simulink model "PhysicalHyperCook"  (R2026b)
settings: Solver=VariableStepAuto  StopTime=14400
undefined symbols (not defined in the file): Fault_T_Cook1, Fault_T_Cook2, Fault_T_Cook3, Fault_T_Cook4, Fault_T_Pack, Fault_T_Prep1, Fault_T_Prep2, Fault_T_QC, HC_PackRate_bph, HC_PrepRate_bph, HC_QCRate_bph, HC_Resupply_bph, Recipe_Block_s, Recipe_Count, Recipe_Flush_s, Resupply_Cutoff_T, Transport_Latency_s, Transport_Rate_bph
(part 2 of 2)

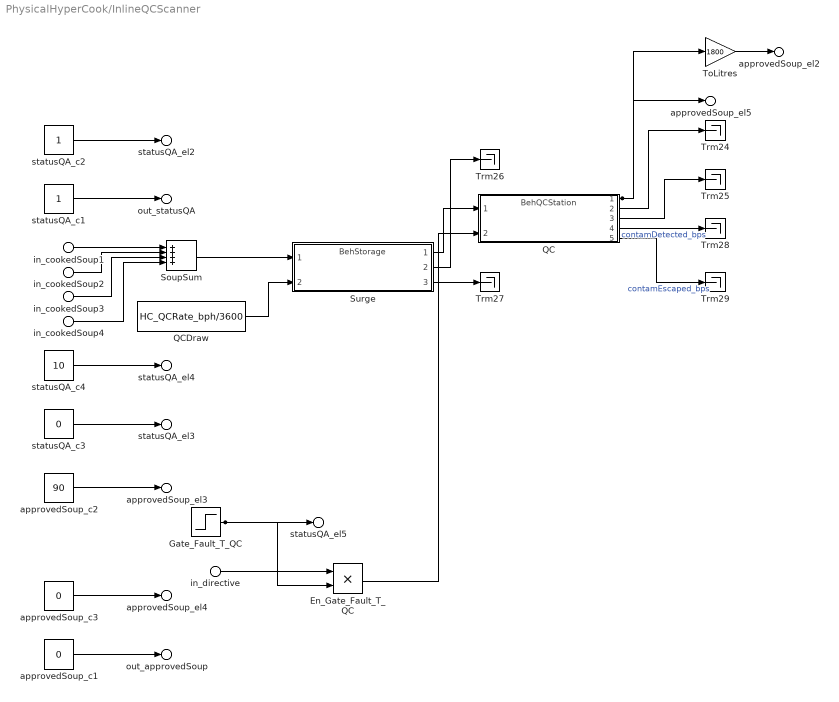
== system PhysicalHyperCook/InlineQCScanner ==
  in_cookedSoup1 : Inport  PortName=cookedSoup1  Element=flow_bps
  in_cookedSoup2 : Inport  Port=2  PortName=cookedSoup2  Element=flow_bps
  in_cookedSoup3 : Inport  Port=3  PortName=cookedSoup3  Element=flow_bps
  in_cookedSoup4 : Inport  Port=4  PortName=cookedSoup4  Element=flow_bps
  in_directive : Inport  Port=5  PortName=directive  Element=setpoint
  En_Gate_Fault_T_QC : Product
  Gate_Fault_T_QC : Step  Time=Fault_T_QC  InitialValue=1  FinalValue=0  SampleTime=0
  QC : ModelReference  ModelNameDialog=BehQCStation  UsingDefaultArgumentValue=0,0,0,0,0,0  SimulationMode=Normal  ModelReferenceVersion=1.6
  QCDraw : Constant  Value=HC_QCRate_bph/3600
  SoupSum : Sum  Inputs=++++
  Surge : ModelReference  ModelNameDialog=BehStorage  UsingDefaultArgumentValue=0,0  SimulationMode=Normal  ModelReferenceVersion=1.4
  ToLitres : Gain  Gain=1800
  Trm{24..29} (6 alike) : Terminator
  approvedSoup_c1 : Constant  Value=0
  approvedSoup_c2 : Constant  Value=90
  approvedSoup_c3 : Constant  Value=0
  statusQA_c1 : Constant
  statusQA_c2 : Constant
  statusQA_c3 : Constant  Value=0
  statusQA_c4 : Constant  Value=10
  out_approvedSoup : Outport  PortName=approvedSoup  Element=batchId
  approvedSoup_el2 : Outport  PortName=approvedSoup  Element=volume_L
  approvedSoup_el3 : Outport  PortName=approvedSoup  Element=temp_C
  approvedSoup_el4 : Outport  PortName=approvedSoup  Element=contamination_ppm
  approvedSoup_el5 : Outport  PortName=approvedSoup  Element=flow_bps
  out_statusQA : Outport  Port=2  PortName=statusQA  Element=unitId
  statusQA_el2 : Outport  Port=2  PortName=statusQA  Element=opState
  statusQA_el3 : Outport  Port=2  PortName=statusQA  Element=faultCode
  statusQA_el4 : Outport  Port=2  PortName=statusQA  Element=power_kW
  statusQA_el5 : Outport  Port=2  PortName=statusQA  Element=health
  wires:
  Surge/1 -> QC/1
  statusQA_c4/1 -> statusQA_el4/1
  QC/3 -> Trm25/1
  statusQA_c2/1 -> statusQA_el2/1
  statusQA_c1/1 -> out_statusQA/1
  ToLitres/1 -> approvedSoup_el2/1
  in_cookedSoup3/1 -> SoupSum/3
  QC/2 -> Trm24/1
  in_cookedSoup1/1 -> SoupSum/1
  in_cookedSoup2/1 -> SoupSum/2
  in_cookedSoup4/1 -> SoupSum/4
  statusQA_c3/1 -> statusQA_el3/1
  approvedSoup_c2/1 -> approvedSoup_el3/1
  approvedSoup_c3/1 -> approvedSoup_el4/1
  approvedSoup_c1/1 -> out_approvedSoup/1
  SoupSum/1 -> Surge/1
  QCDraw/1 -> Surge/2
  Gate_Fault_T_QC/1 -> En_Gate_Fault_T_QC/2, statusQA_el5/1
  in_directive/1 -> En_Gate_Fault_T_QC/1
  Surge/2 -> Trm26/1
  QC/4 -> Trm28/1  "contamDetected_bps"
  Surge/3 -> Trm27/1
  En_Gate_Fault_T_QC/1 -> QC/2
  QC/1 -> approvedSoup_el5/1, ToLitres/1
  QC/5 -> Trm29/1  "contamEscaped_bps"

== system PhysicalHyperCook/InventorySensorGrid ==
  in_stockCold : Inport  PortName=stockCold
  in_stockAmbient : Inport  Port=2  PortName=stockAmbient
  inventoryStatus_c1 : Constant
  inventoryStatus_c2 : Constant  Value=800
  inventoryStatus_c3 : Constant  Value=0
  reorderRequest_c1 : Constant
  reorderRequest_c2 : Constant  Value=0
  reorderRequest_c3 : Constant  Value=0
  out_inventoryStatus : Outport  PortName=inventoryStatus  Element=itemId
  inventoryStatus_el2 : Outport  PortName=inventoryStatus  Element=qty_units
  inventoryStatus_el3 : Outport  PortName=inventoryStatus  Element=error_pct
  out_reorderRequest : Outport  Port=2  PortName=reorderRequest  Element=itemId
  reorderRequest_el2 : Outport  Port=2  PortName=reorderRequest  Element=qty_units
  reorderRequest_el3 : Outport  Port=2  PortName=reorderRequest  Element=error_pct
  wires:
  inventoryStatus_c2/1 -> inventoryStatus_el2/1
  reorderRequest_c2/1 -> reorderRequest_el2/1
  reorderRequest_c3/1 -> reorderRequest_el3/1
  inventoryStatus_c1/1 -> out_inventoryStatus/1
  reorderRequest_c1/1 -> out_reorderRequest/1
  inventoryStatus_c3/1 -> inventoryStatus_el3/1

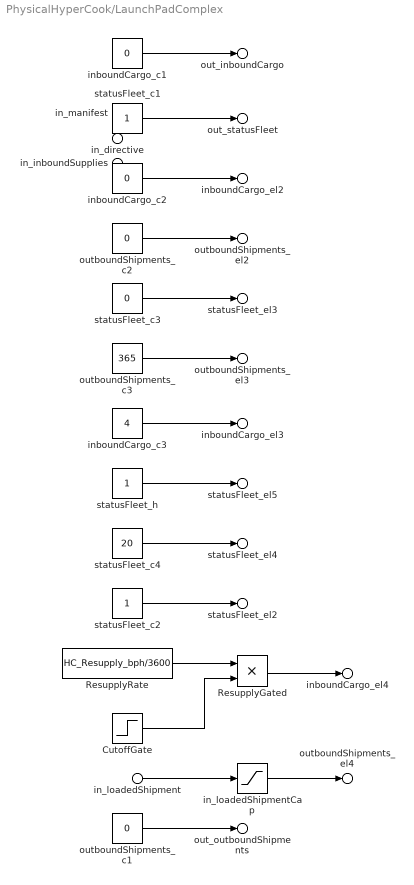
== system PhysicalHyperCook/LaunchPadComplex ==
  in_loadedShipment : Inport  PortName=loadedShipment  Element=flow_bps
  in_manifest : Inport  Port=2  PortName=manifest
  in_directive : Inport  Port=3  PortName=directive
  in_inboundSupplies : Inport  Port=4  PortName=inboundSupplies
  CutoffGate : Step  Time=Resupply_Cutoff_T  InitialValue=1  FinalValue=0  SampleTime=0
  ResupplyGated : Product
  ResupplyRate : Constant  Value=HC_Resupply_bph/3600
  in_loadedShipmentCap : Saturate  UpperLimit=0.1  LowerLimit=0
  inboundCargo_c1 : Constant  Value=0
  inboundCargo_c2 : Constant  Value=0
  inboundCargo_c3 : Constant  Value=4
  outboundShipments_c1 : Constant  Value=0
  outboundShipments_c2 : Constant  Value=0
  outboundShipments_c3 : Constant  Value=365
  statusFleet_c1 : Constant
  statusFleet_c2 : Constant
  statusFleet_c3 : Constant  Value=0
  statusFleet_c4 : Constant  Value=20
  statusFleet_h : Constant
  out_inboundCargo : Outport  PortName=inboundCargo  Element=palletId
  inboundCargo_el2 : Outport  PortName=inboundCargo  Element=mass_kg
  inboundCargo_el3 : Outport  PortName=inboundCargo  Element=temp_C
  inboundCargo_el4 : Outport  PortName=inboundCargo  Element=flow_bps
  out_outboundShipments : Outport  Port=2  PortName=outboundShipments  Element=batchId
  outboundShipments_el2 : Outport  Port=2  PortName=outboundShipments  Element=count
  outboundShipments_el3 : Outport  Port=2  PortName=outboundShipments  Element=sealRating_days
  outboundShipments_el4 : Outport  Port=2  PortName=outboundShipments  Element=flow_bps
  out_statusFleet : Outport  Port=3  PortName=statusFleet  Element=unitId
  statusFleet_el2 : Outport  Port=3  PortName=statusFleet  Element=opState
  statusFleet_el3 : Outport  Port=3  PortName=statusFleet  Element=faultCode
  statusFleet_el4 : Outport  Port=3  PortName=statusFleet  Element=power_kW
  statusFleet_el5 : Outport  Port=3  PortName=statusFleet  Element=health
  wires:
  inboundCargo_c2/1 -> inboundCargo_el2/1
  inboundCargo_c1/1 -> out_inboundCargo/1
  statusFleet_c1/1 -> out_statusFleet/1
  outboundShipments_c2/1 -> outboundShipments_el2/1
  statusFleet_c3/1 -> statusFleet_el3/1
  outboundShipments_c3/1 -> outboundShipments_el3/1
  inboundCargo_c3/1 -> inboundCargo_el3/1
  statusFleet_h/1 -> statusFleet_el5/1
  statusFleet_c4/1 -> statusFleet_el4/1
  statusFleet_c2/1 -> statusFleet_el2/1
  ResupplyRate/1 -> ResupplyGated/1
  CutoffGate/1 -> ResupplyGated/2
  in_loadedShipment/1 -> in_loadedShipmentCap/1
  outboundShipments_c1/1 -> out_outboundShipments/1
  ResupplyGated/1 -> inboundCargo_el4/1
  in_loadedShipmentCap/1 -> outboundShipments_el4/1

== system PhysicalHyperCook/RefuelingStation ==
  in_directive : Inport  PortName=directive
  statusRefuel_c1 : Constant
  statusRefuel_c2 : Constant
  statusRefuel_c3 : Constant  Value=0
  statusRefuel_c4 : Constant  Value=20
  statusRefuel_h : Constant
  out_statusRefuel : Outport  PortName=statusRefuel  Element=unitId
  statusRefuel_el2 : Outport  PortName=statusRefuel  Element=opState
  statusRefuel_el3 : Outport  PortName=statusRefuel  Element=faultCode
  statusRefuel_el4 : Outport  PortName=statusRefuel  Element=power_kW
  statusRefuel_el5 : Outport  PortName=statusRefuel  Element=health
  wires:
  statusRefuel_c1/1 -> out_statusRefuel/1
  statusRefuel_h/1 -> statusRefuel_el5/1
  statusRefuel_c3/1 -> statusRefuel_el3/1
  statusRefuel_c4/1 -> statusRefuel_el4/1
  statusRefuel_c2/1 -> statusRefuel_el2/1

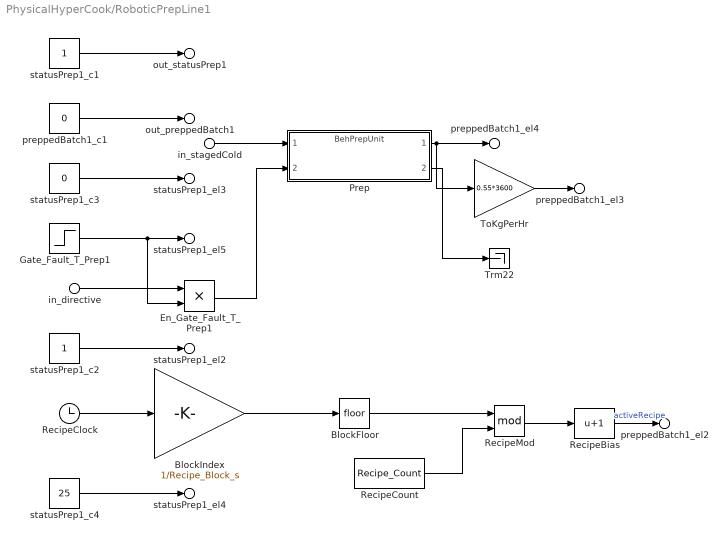
== system PhysicalHyperCook/RoboticPrepLine1 ==
  in_stagedCold : Inport  PortName=stagedCold  Element=flow_bps
  in_directive : Inport  Port=2  PortName=directive  Element=setpoint
  BlockFloor : Rounding
  BlockIndex : Gain  Gain=1/Recipe_Block_s
  En_Gate_Fault_T_Prep1 : Product
  Gate_Fault_T_Prep1 : Step  Time=Fault_T_Prep1  InitialValue=1  FinalValue=0  SampleTime=0
  Prep : ModelReference  ModelNameDialog=BehPrepUnit  UsingDefaultArgumentValue=0,0  SimulationMode=Normal  ModelReferenceVersion=1.5
  RecipeBias : Bias  Bias=1  SaturateOnIntegerOverflow=off
  RecipeClock : Clock
  RecipeCount : Constant  Value=Recipe_Count
  RecipeMod : Math  Operator=mod
  ToKgPerHr : Gain  Gain=0.55*3600
  Trm22 : Terminator
  preppedBatch1_c1 : Constant  Value=0
  statusPrep1_c1 : Constant
  statusPrep1_c2 : Constant
  statusPrep1_c3 : Constant  Value=0
  statusPrep1_c4 : Constant  Value=25
  out_preppedBatch1 : Outport  PortName=preppedBatch1  Element=batchId
  preppedBatch1_el2 : Outport  PortName=preppedBatch1  Element=recipeId
  preppedBatch1_el3 : Outport  PortName=preppedBatch1  Element=mass_kg
  preppedBatch1_el4 : Outport  PortName=preppedBatch1  Element=flow_bps
  out_statusPrep1 : Outport  Port=2  PortName=statusPrep1  Element=unitId
  statusPrep1_el2 : Outport  Port=2  PortName=statusPrep1  Element=opState
  statusPrep1_el3 : Outport  Port=2  PortName=statusPrep1  Element=faultCode
  statusPrep1_el4 : Outport  Port=2  PortName=statusPrep1  Element=power_kW
  statusPrep1_el5 : Outport  Port=2  PortName=statusPrep1  Element=health
  wires:
  statusPrep1_c4/1 -> statusPrep1_el4/1
  statusPrep1_c1/1 -> out_statusPrep1/1
  statusPrep1_c2/1 -> statusPrep1_el2/1
  preppedBatch1_c1/1 -> out_preppedBatch1/1
  statusPrep1_c3/1 -> statusPrep1_el3/1
  in_directive/1 -> En_Gate_Fault_T_Prep1/1
  RecipeClock/1 -> BlockIndex/1
  Gate_Fault_T_Prep1/1 -> En_Gate_Fault_T_Prep1/2, statusPrep1_el5/1
  RecipeCount/1 -> RecipeMod/2
  in_stagedCold/1 -> Prep/1
  En_Gate_Fault_T_Prep1/1 -> Prep/2
  BlockIndex/1 -> BlockFloor/1
  Prep/1 -> ToKgPerHr/1, preppedBatch1_el4/1
  Prep/2 -> Trm22/1
  BlockFloor/1 -> RecipeMod/1
  ToKgPerHr/1 -> preppedBatch1_el3/1
  RecipeMod/1 -> RecipeBias/1
  RecipeBias/1 -> preppedBatch1_el2/1  "activeRecipe"

== system PhysicalHyperCook/RoboticPrepLine2 ==
  in_stagedAmbient : Inport  PortName=stagedAmbient  Element=flow_bps
  in_directive : Inport  Port=2  PortName=directive  Element=setpoint
  BlockFloor : Rounding
  BlockIndex : Gain  Gain=1/Recipe_Block_s
  En_Gate_Fault_T_Prep2 : Product
  Gate_Fault_T_Prep2 : Step  Time=Fault_T_Prep2  InitialValue=1  FinalValue=0  SampleTime=0
  Prep : ModelReference  ModelNameDialog=BehPrepUnit  UsingDefaultArgumentValue=0,0  SimulationMode=Normal  ModelReferenceVersion=1.5
  RecipeBias : Bias  Bias=1  SaturateOnIntegerOverflow=off
  RecipeClock : Clock
  RecipeCount : Constant  Value=Recipe_Count
  RecipeMod : Math  Operator=mod
  ToKgPerHr : Gain  Gain=0.55*3600
  Trm23 : Terminator
  preppedBatch2_c1 : Constant  Value=0
  statusPrep2_c1 : Constant
  statusPrep2_c2 : Constant
  statusPrep2_c3 : Constant  Value=0
  statusPrep2_c4 : Constant  Value=25
  out_preppedBatch2 : Outport  PortName=preppedBatch2  Element=batchId
  preppedBatch2_el2 : Outport  PortName=preppedBatch2  Element=recipeId
  preppedBatch2_el3 : Outport  PortName=preppedBatch2  Element=mass_kg
  preppedBatch2_el4 : Outport  PortName=preppedBatch2  Element=flow_bps
  out_statusPrep2 : Outport  Port=2  PortName=statusPrep2  Element=unitId
  statusPrep2_el2 : Outport  Port=2  PortName=statusPrep2  Element=opState
  statusPrep2_el3 : Outport  Port=2  PortName=statusPrep2  Element=faultCode
  statusPrep2_el4 : Outport  Port=2  PortName=statusPrep2  Element=power_kW
  statusPrep2_el5 : Outport  Port=2  PortName=statusPrep2  Element=health
  wires:
  statusPrep2_c1/1 -> out_statusPrep2/1
  statusPrep2_c3/1 -> statusPrep2_el3/1
  RecipeClock/1 -> BlockIndex/1
  RecipeBias/1 -> preppedBatch2_el2/1
  preppedBatch2_c1/1 -> out_preppedBatch2/1
  BlockIndex/1 -> BlockFloor/1
  statusPrep2_c2/1 -> statusPrep2_el2/1
  Gate_Fault_T_Prep2/1 -> En_Gate_Fault_T_Prep2/2, statusPrep2_el5/1
  statusPrep2_c4/1 -> statusPrep2_el4/1
  in_directive/1 -> En_Gate_Fault_T_Prep2/1
  in_stagedAmbient/1 -> Prep/1
  En_Gate_Fault_T_Prep2/1 -> Prep/2
  Prep/1 -> preppedBatch2_el4/1, ToKgPerHr/1
  Prep/2 -> Trm23/1
  BlockFloor/1 -> RecipeMod/1
  RecipeCount/1 -> RecipeMod/2
  ToKgPerHr/1 -> preppedBatch2_el3/1
  RecipeMod/1 -> RecipeBias/1
